simulink model "finalSim"  (R2022b)
settings: Solver=VariableStepAuto  StartTime=0.0  StopTime=10.0  RelTol=1e-3
values from neighbouring files (symbols this model uses):
  k = par(1)    [finalScript.m]
  t_m = par(2)    [finalScript.m]
  U_pr = vols(i)    [finalScript.m]
settings Model: Creator=kladm  LastModifiedBy=skifp

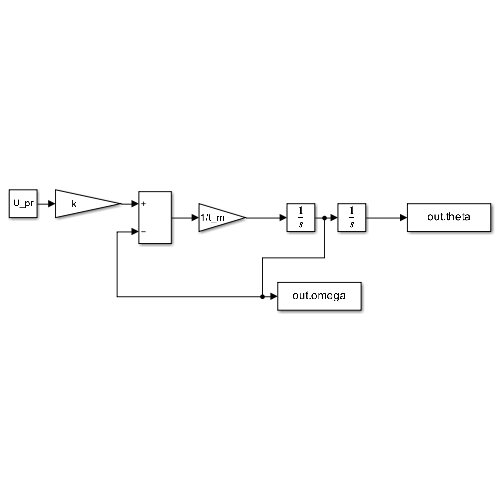
[thumbnail: Simulink's stored preview of the top-level diagram]
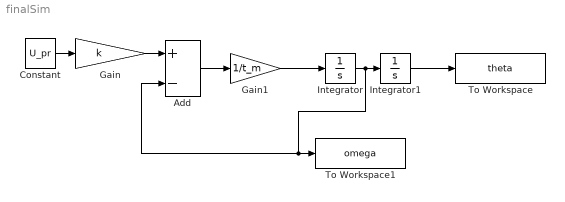
== system finalSim ==
  Add : Sum  Inputs=+-
  Constant : Constant  Value=U_pr
  Gain : Gain  Gain=k
  Gain1 : Gain  Gain=1/t_m
  Integrator : Integrator
  Integrator1 : Integrator
  To Workspace : ToWorkspace  VariableName=theta  SaveFormat=Timeseries  SampleTime=-1
  To Workspace1 : ToWorkspace  VariableName=omega  SaveFormat=Timeseries  SampleTime=-1
  wires:
  Constant/1 -> Gain/1
  Gain/1 -> Add/1
  Add/1 -> Gain1/1
  Gain1/1 -> Integrator/1
  Integrator/1 -> To Workspace1/1, Add/2, Integrator1/1
  Integrator1/1 -> To Workspace/1
